simulink model "PID_Sim"  (R2020b)
settings: Solver=FixedStepAuto  StartTime=0.0  StopTime=2500.0  FixedStep=1  RelTol=1e-3
values from neighbouring files (symbols this model uses):
  a = a(NNL(i)*NNL(j)+1:end)    [ArrayToCell.m]    (also in CellToArray.m = [a;w2{i,j}(:)]; SelfBuildingNeuralNet.m = [0.5 , 0.7])
  BS = 0    [SelfBuildingNeuralNet.m]
  NI = Net1{1}(1)    [CreateChildren.m]    (also in GetReadyForBackpropagation.m = Data(1); SelfBuildingNeuralNet.m = 1)
  NL = 1    [GetReadyForBackpropagation.m]
  NNL = NO    [GetReadyForBackpropagation.m]
  ymax = max(y)    [GetRedyToUse.m]
  ymin = min(y)    [GetRedyToUse.m]
undefined symbols (not defined in the file or in its folder): wa
libraries: pid_lib x1
settings Model: Creator=varga  LastModifiedBy=varga
settings OptimizationCC: BlockReduction=off  ConditionallyExecuteInputs=off

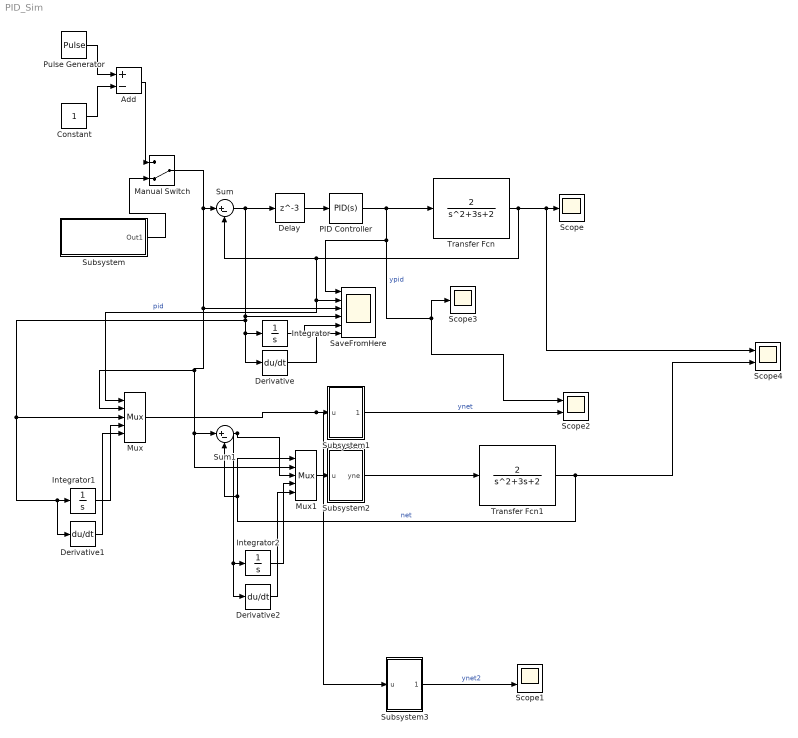
== system PID_Sim ==
  Add : Sum  Inputs=+-
  Constant : Constant
  Delay : Delay  DelayLength=3  InitialCondition=0
  Derivative : Derivative
  Derivative1 : Derivative
  Derivative2 : Derivative
  Integrator : Integrator
  Integrator1 : Integrator
  Integrator2 : Integrator
  Manual Switch : ManualSwitch  CurrentSetting=0
  Mux : Mux  Inputs=5
  Mux1 : Mux  Inputs=5
  PID Controller : pid_lib/PID Controller  Controller=PID  Form=Ideal  TimeDomain=Continuous-time  UseExternalTs=off  SampleTime=-1  IntegratorMethod=Forward Euler  FilterMethod=Forward Euler  ControllerParametersSource=internal  P=0.300434374912646  I=0.579433661057263  D=0  UseFilter=on  N=100  TunerSelectOption=Transfer Function Based (PID Tuner App)  InitialConditionSource=internal  InitialConditionForIntegrator=0  InitialConditionForFilter=0  DifferentiatorICPrevScaledInput=0  ExternalReset=none  TrackingMode=off  Kt=1  LimitOutput=off  SatLimitsSource=internal  UpperSaturationLimit=inf  LowerSaturationLimit=-inf  LinearizeAsGain=on  AntiWindupMode=none  Kb=1  POutMin=[]  POutMax=[]  IOutMin=[]  IOutMax=[]  DOutMin=[]  DOutMax=[]  NOutMin=[]  NOutMax=[]  SumOutMin=[]  SumOutMax=[]  SaturationOutMin=[]  SaturationOutMax=[]  PParamMin=[]  PParamMax=[]  IParamMin=[]  IParamMax=[]  DParamMin=[]  DParamMax=[]  NParamMin=[]  NParamMax=[]  KbParamMin=[]  KbParamMax=[]  KtParamMin=[]  KtParamMax=[]  KbOutMin=[]  KbOutMax=[]  KtOutMin=[]  KtOutMax=[]  IntegratorOutMin=[]  IntegratorOutMax=[]  FilterOutMin=[]  FilterOutMax=[]  SumI1OutMin=[]  SumI1OutMax=[]  SumI2OutMin=[]  SumI2OutMax=[]  SumI3OutMin=[]  SumI3OutMax=[]  SumI4OutMin=[]  SumI4OutMax=[]  SumDOutMin=[]  SumDOutMax=[]  DifferentiatorOutMin=[]  DifferentiatorOutMax=[]  FilterDiffOutCoefMin=[]  FilterDiffOutCoefMax=[]  ReciprocalOutMin=[]  ReciprocalOutMax=[]  SumDenOutMin=[]  SumDenOutMax=[]  SumNumOutMin=[]  SumNumOutMax=[]  DivideOutMin=[]  DivideOutMax=[]  UdiffTsProdOutMin=[]  UdiffTsProdOutMax=[]  NTsProdOutMin=[]  NTsProdOutMax=[]  UintegralTsProdOutMin=[]  UintegralTsProdOutMax=[]  UngainTsProdOutMin=[]  UngainTsProdOutMax=[]  IntegratorContinuousStateAttributes=''  IntegratorStateMustResolveToSignalObject=off  IntegratorRTWStateStorageClass=Auto  FilterContinuousStateAttributes=''  FilterStateMustResolveToSignalObject=off  FilterRTWStateStorageClass=Auto  ParallelPVariant=Passthrough  IdealPVariant=InternalParameters  IVariant=InternalParameters  DVariant=InternalParameters  IntegratorVariant=Continuous  SatVariant=Disabled  AWVariant=Passthrough  PCopyVariant=Disabled  TRVariant=Disabled  FdbkBlocksVariant=Forward  IdealPFdbkVariant=Disabled  SatFdbkVariant=Disabled  DerivativeFilterVariant=ContFilter  NVariant=InternalParameters  NCopyVariant=Disabled  FilterICVariant=InternalICsFilter  IntegratorICVariant=InternalICs  ExternalResetVariant=Disabled  TRSumVariant=Passthrough  SumFdbkVariant=Disabled  SumVariant=Sum_PID  TsampFilterVariant=InternalTs  TsampNgainVariant=Passthrough  TsampIntegralVariant=Passthrough  ExternalSaturationOutDataTypeStr=Inherit: Same as second input
  Pulse Generator : DiscretePulseGenerator  PulseType=Time based  Amplitude=[2]  Period=90  PulseWidth=50
  SaveFromHere : Scope  NumInputPorts=6
  Scope : Scope
  Scope1 : Scope  NumInputPorts=2
  Scope2 : Scope  NumInputPorts=2
  Scope3 : Scope
  Scope4 : Scope  NumInputPorts=2
  Subsystem : Subsystem
  Subsystem1 : Subsystem
  Subsystem2 : Subsystem
  Subsystem3 : Subsystem
  Sum : Sum  Inputs=|+-
  Sum1 : Sum  Inputs=|+-
  Transfer Fcn : TransferFcn  Numerator=[2]  Denominator=[1 3 2]
  Transfer Fcn1 : TransferFcn  Numerator=[2]  Denominator=[1 3 2]
  wires:
  Transfer Fcn/1 -> Mux/1, SaveFromHere/2, Sum/2, Scope4/1, Scope/1  "pid"
  Manual Switch/1 -> Mux1/2, Sum1/1, Mux/2, SaveFromHere/3, Sum/1
  PID Controller/1 -> Scope3/1, Scope2/1, SaveFromHere/1, Transfer Fcn/1  "ypid"
  Delay/1 -> PID Controller/1
  Transfer Fcn1/1 -> Mux1/1, Sum1/2, Scope4/2  "net"
  Constant/1 -> Add/2
  Pulse Generator/1 -> Add/1
  Subsystem/1(Out1) -> Manual Switch/2
  Mux/1 -> Subsystem3/1(u), Subsystem1/1(u)
  Subsystem1/1(ynet) -> Scope2/2  "ynet"
  Subsystem2/1(yne) -> Transfer Fcn1/1
  Mux1/1 -> Subsystem2/1(u)
  Sum1/1 -> Mux1/3, Derivative2/1, Integrator2/1
  Sum/1 -> Derivative1/1, Integrator1/1, Mux/3, Derivative/1, Integrator/1, SaveFromHere/4, Delay/1
  Integrator/1 -> SaveFromHere/5
  Integrator1/1 -> Mux/4
  Integrator2/1 -> Mux1/4
  Derivative/1 -> SaveFromHere/6
  Derivative1/1 -> Mux/5
  Derivative2/1 -> Mux1/5
  Add/1 -> Manual Switch/1
  Subsystem3/1(ynet) -> Scope1/2  "ynet2"

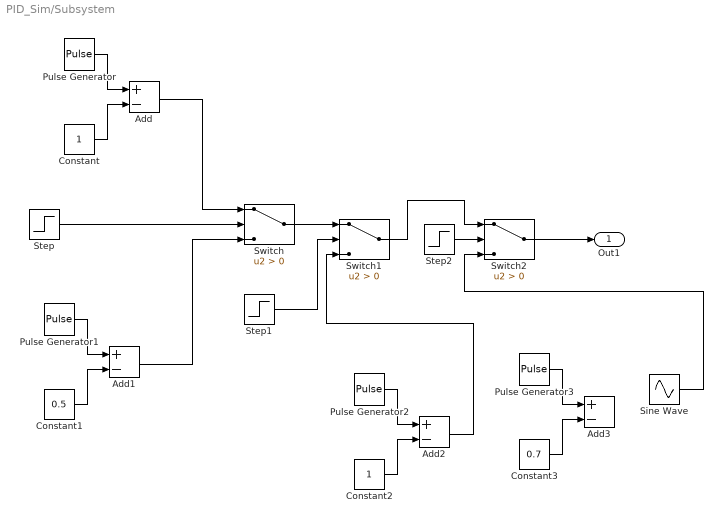
== system PID_Sim/Subsystem ==
  Add{,1..3} (4 alike) : Sum  Inputs=+-
  Constant : Constant
  Constant1 : Constant  Value=0.5
  Constant2 : Constant
  Constant3 : Constant  Value=0.7
  Pulse Generator : DiscretePulseGenerator  PulseType=Time based  Amplitude=[2]  Period=200  PulseWidth=50
  Pulse Generator1 : DiscretePulseGenerator  PulseType=Time based  Amplitude=[1]  Period=140  PulseWidth=50
  Pulse Generator2 : DiscretePulseGenerator  PulseType=Time based  Amplitude=[2]  Period=110  PulseWidth=50
  Pulse Generator3 : DiscretePulseGenerator  PulseType=Time based  Amplitude=[1.4]  Period=90  PulseWidth=50
  Sine Wave : Sin  Frequency=0.2  SampleTime=0
  Step : Step  Time=500  Before=1  After=0  SampleTime=0
  Step1 : Step  Time=1500  Before=1  After=0  SampleTime=0
  Step2 : Step  Time=2100  Before=1  After=0  SampleTime=0
  Switch : Switch  Criteria=u2 > Threshold
  Switch1 : Switch  Criteria=u2 > Threshold
  Switch2 : Switch  Criteria=u2 > Threshold
  Out1 : Outport
  wires:
  Pulse Generator/1 -> Add/1
  Constant/1 -> Add/2
  Add/1 -> Switch/1
  Step/1 -> Switch/2
  Constant1/1 -> Add1/2
  Pulse Generator1/1 -> Add1/1
  Add1/1 -> Switch/3
  Switch/1 -> Switch1/1
  Step1/1 -> Switch1/2
  Constant2/1 -> Add2/2
  Pulse Generator2/1 -> Add2/1
  Add2/1 -> Switch1/3
  Step2/1 -> Switch2/2
  Constant3/1 -> Add3/2
  Pulse Generator3/1 -> Add3/1
  Switch1/1 -> Switch2/1
  Switch2/1 -> Out1/1
  Sine Wave/1 -> Switch2/3

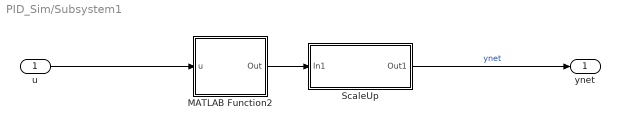
== system PID_Sim/Subsystem1 ==
  u : Inport
  MATLAB Function2 : MATLAB Function  TreatAsAtomicUnit=on  mask{wa=wa, NL=NL, NNL=NNL, NI=NI, NO=0, a=a, BiginnerState=BS}
  ScaleUp : Subsystem  mask{ymax=ymax, ymin=ymin}
  ynet : Outport
  wires:
  u/1 -> MATLAB Function2/1(u)
  MATLAB Function2/1(Out) -> ScaleUp/1(In1)
  ScaleUp/1(Out1) -> ynet/1  "ynet"

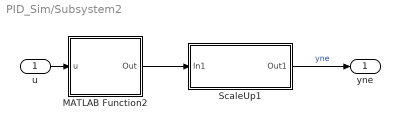
== system PID_Sim/Subsystem2 ==
  u : Inport
  MATLAB Function2 : MATLAB Function  TreatAsAtomicUnit=on  mask{wa=wa, NL=NL, NNL=NNL, NI=NI, NO=0, a=a, BiginnerState=BS}
  ScaleUp1 : Subsystem  mask{ymax=ymax, ymin=ymin}
  yne : Outport
  wires:
  u/1 -> MATLAB Function2/1(u)
  MATLAB Function2/1(Out) -> ScaleUp1/1(In1)
  ScaleUp1/1(Out1) -> yne/1  "yne"

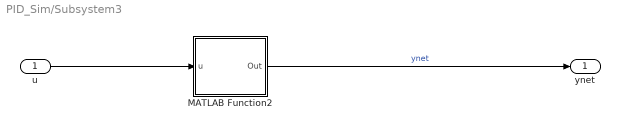
== system PID_Sim/Subsystem3 ==
  u : Inport
  MATLAB Function2 : MATLAB Function  TreatAsAtomicUnit=on  mask{wa=wa, NL=NL, NNL=NNL, NI=NI, NO=0, a=a, BiginnerState=BS}
  ynet : Outport
  wires:
  u/1 -> MATLAB Function2/1(u)
  MATLAB Function2/1(Out) -> ynet/1  "ynet"

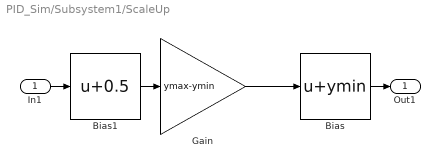
== system PID_Sim/Subsystem1/ScaleUp ==
  In1 : Inport
  Bias : Bias  Bias=ymin
  Bias1 : Bias  Bias=0.5
  Gain : Gain  Gain=ymax-ymin
  Out1 : Outport
  wires:
  Gain/1 -> Bias/1
  In1/1 -> Bias1/1
  Bias/1 -> Out1/1
  Bias1/1 -> Gain/1

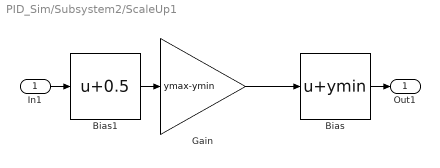
== system PID_Sim/Subsystem2/ScaleUp1 ==
  In1 : Inport
  Bias : Bias  Bias=ymin
  Bias1 : Bias  Bias=0.5
  Gain : Gain  Gain=ymax-ymin
  Out1 : Outport
  wires:
  Gain/1 -> Bias/1
  In1/1 -> Bias1/1
  Bias/1 -> Out1/1
  Bias1/1 -> Gain/1

== matlab function PID_Sim/Subsystem2/MATLAB Function2 ==
  settings: updateMethod=DISCRETE
  data: u input; Out output size=1; wa parameter; NL parameter; NNL parameter; a parameter; BiginnerState parameter; NI parameter; NO parameter
function Out = fcn(u,wa,NL, NNL,a, BiginnerState, NI,NO)
[n,m]=size(u);
w=cell(1,2);
w=ArrayToCell(wa,NL,NNL,NI);

w1 = w{1};
w2 = w{2};
NLI=[NI,NNL];

persistent y;
if isempty(y)
    y=cell(1,NL);
    for i=1:NL
    y{i}=zeros(NNL(i),1)+BiginnerState; %hányadik réteg, hányadik kimenet
    % minden réteg kimenetét beállítom a kezdeti értékre
    end
end

persistent x;
if isempty(x)
    NIL=NL+1;
    x=cell(1,NIL);
    
    
    for i=1:NIL
      %  x{j}=[1;y{j-1}];
        x{i}=[1;zeros(NLI(i),1)+BiginnerState];
    % minden réteg bemenetét beállítom a kezdeti értékre
    end
end

persistent s1;
if isempty(s1)
    s1=cell(1,NL); 
    for j=1:NL     
        s1{j}=zeros(NNL(j),1);
    end
end

persistent s2;
if isempty(s2)
    s2=cell(1,NL); 
    for j=1:NL     
        s2{j}=zeros(NNL(j),1);
    end
end

persistent s;
if isempty(s)
    s=cell(1,NL); 
    for j=1:NL     
        s{j}=zeros(NNL(j),1);
    end
end


x{1}=[1;u];                    %az adottt layer elorecstolt bemenete

for j=2:NL+1     
        x{j}=[1;y{j-1}];
end

for j=1:NL
        s1{j}=w1{j}*x{1};   % s{j} oszlop
       
        s2{j}=zeros(NNL(j),1);
        
        for k=j:NL
            s2{j}=s2{j}+ w2{j,k}*x{k+1}(2:length(x{k+1}),:);  
        end    
        
        s{j}=s1{j}+s2{j};
    
end

    for j=1:NL
        
        k=zeros(NNL(j),1);
        z=ActFunc(s{:,j},a)
        k(1:NNL(j),1)=z(1:NNL(j),1);
        y{j}=k;
        
    end



    
Out=y{end}(1);

end



function y=ActFunc(s,a)
    teta=0;
   y=(1-exp(-(a*s-teta)))./(1+exp(-(a*s-teta)));
end

function w = ArrayToCell(a,NL,NNL,NI)


w1=cell(1,NL);
w2=cell(NL,NL);
w=cell(1,2);
a0=1;

for i=1:NL
    
    w1{i}=reshape(a(a0:a0-1+NNL(i)*(NI+1)),NNL(i),NI+1);
    a0=a0+NNL(i)*(NI+1);
    
    
end

for i=1:NL
    for j=1:NL
        w2{i,j}=reshape(a(a0:a0-1+NNL(i)*NNL(j)),NNL(i),NNL(j));
        a0=a0+NNL(i)*NNL(j);
    end
end

w={w1,w2};

end

== matlab function PID_Sim/Subsystem1/MATLAB Function2 ==
  settings: updateMethod=DISCRETE
  data: u input; Out output size=1; wa parameter; NL parameter; NNL parameter; a parameter; BiginnerState parameter; NI parameter; NO parameter
function Out = fcn(u,wa,NL, NNL,a, BiginnerState, NI,NO)
[n,m]=size(u);
w=cell(1,2);
w=ArrayToCell(wa,NL,NNL,NI);

w1 = w{1};
w2 = w{2};
NLI=[NI,NNL];

persistent y;
if isempty(y)
    y=cell(1,NL);
    for i=1:NL
    y{i}=zeros(NNL(i),1)+BiginnerState; %hányadik réteg, hányadik kimenet
    % minden réteg kimenetét beállítom a kezdeti értékre
    end
end

persistent x;
if isempty(x)
    NIL=NL+1;
    x=cell(1,NIL);
    
    
    for i=1:NIL
      %  x{j}=[1;y{j-1}];
        x{i}=[1;zeros(NLI(i),1)+BiginnerState];
    % minden réteg bemenetét beállítom a kezdeti értékre
    end
end

persistent s1;
if isempty(s1)
    s1=cell(1,NL); 
    for j=1:NL     
        s1{j}=zeros(NNL(j),1);
    end
end

persistent s2;
if isempty(s2)
    s2=cell(1,NL); 
    for j=1:NL     
        s2{j}=zeros(NNL(j),1);
    end
end

persistent s;
if isempty(s)
    s=cell(1,NL); 
    for j=1:NL     
        s{j}=zeros(NNL(j),1);
    end
end


x{1}=[1;u];                    %az adottt layer elorecstolt bemenete

for j=2:NL+1     
        x{j}=[1;y{j-1}];
end

for j=1:NL
        s1{j}=w1{j}*x{1};   % s{j} oszlop
       
        s2{j}=zeros(NNL(j),1);
        
        for k=j:NL
            s2{j}=s2{j}+ w2{j,k}*x{k+1}(2:length(x{k+1}),:);  
        end    
        
        s{j}=s1{j}+s2{j};
    
end

    for j=1:NL
        
        k=zeros(NNL(j),1);
        z=ActFunc(s{:,j},a)
        k(1:NNL(j),1)=z(1:NNL(j),1);
        y{j}=k;
        
    end



    
Out=y{end}(1);

end



function y=ActFunc(s,a)
    teta=0;
   y=(1-exp(-(a*s-teta)))./(1+exp(-(a*s-teta)));
end

function w = ArrayToCell(a,NL,NNL,NI)


w1=cell(1,NL);
w2=cell(NL,NL);
w=cell(1,2);
a0=1;

for i=1:NL
    
    w1{i}=reshape(a(a0:a0-1+NNL(i)*(NI+1)),NNL(i),NI+1);
    a0=a0+NNL(i)*(NI+1);
    
    
end

for i=1:NL
    for j=1:NL
        w2{i,j}=reshape(a(a0:a0-1+NNL(i)*NNL(j)),NNL(i),NNL(j));
        a0=a0+NNL(i)*NNL(j);
    end
end

w={w1,w2};

end

== matlab function PID_Sim/Subsystem3/MATLAB Function2 ==
  settings: updateMethod=DISCRETE
  data: u input; Out output size=1; wa parameter; NL parameter; NNL parameter; a parameter; BiginnerState parameter; NI parameter; NO parameter
function Out = fcn(u,wa,NL, NNL,a, BiginnerState, NI,NO)
[n,m]=size(u);
w=cell(1,2);
w=ArrayToCell(wa,NL,NNL,NI);

w1 = w{1};
w2 = w{2};
NLI=[NI,NNL];

persistent y;
if isempty(y)
    y=cell(1,NL);
    for i=1:NL
    y{i}=zeros(NNL(i),1)+BiginnerState; %hányadik réteg, hányadik kimenet
    % minden réteg kimenetét beállítom a kezdeti értékre
    end
end

persistent x;
if isempty(x)
    NIL=NL+1;
    x=cell(1,NIL);
    
    
    for i=1:NIL
      %  x{j}=[1;y{j-1}];
        x{i}=[1;zeros(NLI(i),1)+BiginnerState];
    % minden réteg bemenetét beállítom a kezdeti értékre
    end
end

persistent s1;
if isempty(s1)
    s1=cell(1,NL); 
    for j=1:NL     
        s1{j}=zeros(NNL(j),1);
    end
end

persistent s2;
if isempty(s2)
    s2=cell(1,NL); 
    for j=1:NL     
        s2{j}=zeros(NNL(j),1);
    end
end

persistent s;
if isempty(s)
    s=cell(1,NL); 
    for j=1:NL     
        s{j}=zeros(NNL(j),1);
    end
end


x{1}=[1;u];                    %az adottt layer elorecstolt bemenete

for j=2:NL+1     
        x{j}=[1;y{j-1}];
end

for j=1:NL
        s1{j}=w1{j}*x{1};   % s{j} oszlop
       
        s2{j}=zeros(NNL(j),1);
        
        for k=j:NL
            s2{j}=s2{j}+ w2{j,k}*x{k+1}(2:length(x{k+1}),:);  
        end    
        
        s{j}=s1{j}+s2{j};
    
end

    for j=1:NL
        
        k=zeros(NNL(j),1);
        z=ActFunc(s{:,j},a)
        k(1:NNL(j),1)=z(1:NNL(j),1);
        y{j}=k;
        
    end



    
Out=y{end}(1);

end



function y=ActFunc(s,a)
    teta=0;
   y=(1-exp(-(a*s-teta)))./(1+exp(-(a*s-teta)));
end

function w = ArrayToCell(a,NL,NNL,NI)


w1=cell(1,NL);
w2=cell(NL,NL);
w=cell(1,2);
a0=1;

for i=1:NL
    
    w1{i}=reshape(a(a0:a0-1+NNL(i)*(NI+1)),NNL(i),NI+1);
    a0=a0+NNL(i)*(NI+1);
    
    
end

for i=1:NL
    for j=1:NL
        w2{i,j}=reshape(a(a0:a0-1+NNL(i)*NNL(j)),NNL(i),NNL(j));
        a0=a0+NNL(i)*NNL(j);
    end
end

w={w1,w2};

end
